simulink model "soru2d2"  (R2019a)
settings: Solver=VariableStepAuto  StartTime=0.0  StopTime=1000  RelTol=1e-3
settings Model: Creator=handeyildirim  LastModifiedBy=handeyildirim

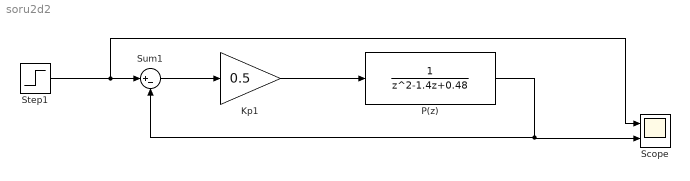
== system soru2d2 ==
  Kp1 : Gain  Gain=0.5
  P(z) : DiscreteTransferFcn  Denominator=[1 -1.4 0.48]  SampleTime=1
  Scope : Scope  NumInputPorts=2
  Step1 : Step  SampleTime=1
  Sum1 : Sum  Inputs=|+-
  wires:
  Step1/1 -> Scope/1, Sum1/1
  P(z)/1 -> Scope/2, Sum1/2
  Kp1/1 -> P(z)/1
  Sum1/1 -> Kp1/1
